simulink model "twoaxis_camera_gantry_start_work_project_Yejesh_final"  (R2025b)
settings: Solver=ode15s  StartTime=0.0  StopTime=60  MaxStep=1e-3  RelTol=1e-3  EnableMultiTasking=on
model workspace: external: MATLAB File gantryParams.m (data not in the file)
undefined symbols (not defined in the file): endSupport, endSupportZ, fractalcoef, leadScrew, leadScrewZ, rail, railZ, runner, runnerZ, X, Y, Z
libraries: sm_lib x81, nesl_utility x14, sm_linear_actuator_lib x14, fl_lib x6, slpidlib x2, mspsensorlib x1
(part 2 of 4)

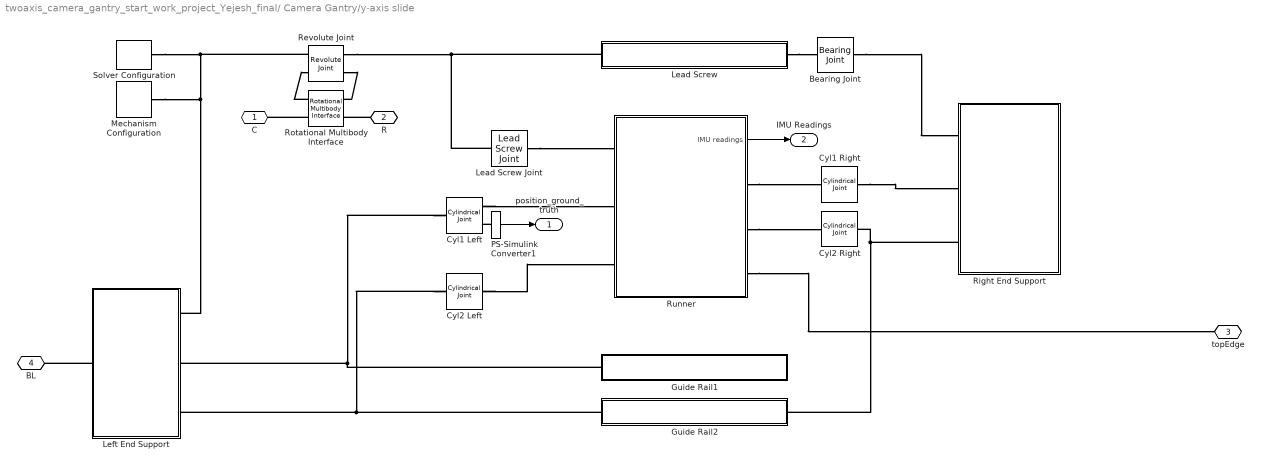
== system twoaxis_camera_gantry_start_work_project_Yejesh_final/	Camera Gantry/y-axis slide ==
  Bearing Joint : sm_lib/Joints/Bearing Joint  StatePerturbationForJacobian=1.0e-05  JointMode=Normal  CompositeWrenchDir=FollowerOnBase  CompositeWrenchFrame=BaseFrame  SenseConstraintForce=off  SenseConstraintTorque=off  SenseTotalForce=off  SenseTotalTorque=off  PzPositionTargetSpecify=off  PzPositionTargetPriority=High  PzPositionTargetValue=0  PzPositionTargetValueUnits=m  PzVelocityTargetSpecify=off  PzVelocityTargetPriority=High  PzVelocityTargetValue=0  PzVelocityTargetValueUnits=m/s  PzEquilibriumPosition=0  PzEquilibriumPositionUnits=m  PzSpringStiffness=0  PzSpringStiffnessUnits=N/m  PzDampingCoefficient=0  PzDampingCoefficientUnits=N/(m/s)  PzLowerLimitSpecify=off  PzLowerLimitBound=-1  PzLowerLimitBoundUnits=m  PzLowerLimitStiffness=1e6  PzLowerLimitStiffnessUnits=N/m  PzLowerLimitDamping=1e3  PzLowerLimitDampingUnits=N/(m/s)  PzLowerLimitTransitionRegionWidth=1e-4  PzLowerLimitTransitionRegionWidthUnits=m  PzUpperLimitSpecify=off  PzUpperLimitBound=1  PzUpperLimitBoundUnits=m  PzUpperLimitStiffness=1e6  PzUpperLimitStiffnessUnits=N/m  PzUpperLimitDamping=1e3  PzUpperLimitDampingUnits=N/(m/s)  PzUpperLimitTransitionRegionWidth=1e-4  PzUpperLimitTransitionRegionWidthUnits=m  PzTorqueActuationMode=NoTorque  PzMotionActuationMode=ComputedMotion  PzSensePosition=off  PzSenseVelocity=off  PzSenseAcceleration=off  PzSenseTorqueForce=off  PzSenseLowerLimitTorqueForce=off  PzSenseUpperLimitTorqueForce=off  RxPositionTargetSpecify=off  RxPositionTargetPriority=High  RxPositionTargetValue=0  RxPositionTargetValueUnits=deg  RxVelocityTargetSpecify=off  RxVelocityTargetPriority=High  RxVelocityTargetValue=0  RxVelocityTargetValueUnits=deg/s  RxEquilibriumPosition=0  RxEquilibriumPositionUnits=deg  RxSpringStiffness=0  RxSpringStiffnessUnits=N*m/deg  RxDampingCoefficient=0  RxDampingCoefficientUnits=N*m/(deg/s)  RxLowerLimitSpecify=off  RxLowerLimitBound=-90  RxLowerLimitBoundUnits=deg  RxLowerLimitStiffness=1e4  RxLowerLimitStiffnessUnits=N*m/deg  RxLowerLimitDamping=10  RxLowerLimitDampingUnits=N*m/(deg/s)  RxLowerLimitTransitionRegionWidth=0.1  RxLowerLimitTransitionRegionWidthUnits=deg  RxUpperLimitSpecify=off  RxUpperLimitBound=90  RxUpperLimitBoundUnits=deg  RxUpperLimitStiffness=1e4  RxUpperLimitStiffnessUnits=N*m/deg  RxUpperLimitDamping=10  RxUpperLimitDampingUnits=N*m/(deg/s)  RxUpperLimitTransitionRegionWidth=0.1  RxUpperLimitTransitionRegionWidthUnits=deg  RxTorqueActuationMode=NoTorque  RxMotionActuationMode=ComputedMotion  RxSensePosition=off  RxSenseVelocity=off  RxSenseAcceleration=off  RxSenseTorqueForce=off  RxSenseLowerLimitTorqueForce=off  RxSenseUpperLimitTorqueForce=off  RyPositionTargetSpecify=off  RyPositionTargetPriority=High  RyPositionTargetValue=0  RyPositionTargetValueUnits=deg  RyVelocityTargetSpecify=off  RyVelocityTargetPriority=High  RyVelocityTargetValue=0  RyVelocityTargetValueUnits=deg/s  RyEquilibriumPosition=0  RyEquilibriumPositionUnits=deg  RySpringStiffness=0  RySpringStiffnessUnits=N*m/deg  RyDampingCoefficient=0  RyDampingCoefficientUnits=N*m/(deg/s)  RyLowerLimitSpecify=off  RyLowerLimitBound=-90  RyLowerLimitBoundUnits=deg  RyLowerLimitStiffness=1e4  RyLowerLimitStiffnessUnits=N*m/deg  RyLowerLimitDamping=10  RyLowerLimitDampingUnits=N*m/(deg/s)  RyLowerLimitTransitionRegionWidth=0.1  RyLowerLimitTransitionRegionWidthUnits=deg  RyUpperLimitSpecify=off  RyUpperLimitBound=90  RyUpperLimitBoundUnits=deg  RyUpperLimitStiffness=1e4  RyUpperLimitStiffnessUnits=N*m/deg  RyUpperLimitDamping=10  RyUpperLimitDampingUnits=N*m/(deg/s)  RyUpperLimitTransitionRegionWidth=0.1  RyUpperLimitTransitionRegionWidthUnits=deg  RyTorqueActuationMode=NoTorque  RyMotionActuationMode=ComputedMotion  RySensePosition=off  RySenseVelocity=off  RySenseAcceleration=off  RySenseTorqueForce=off  RySenseLowerLimitTorqueForce=off  RySenseUpperLimitTorqueForce=off  RzPositionTargetSpecify=off  RzPositionTargetPriority=High  RzPositionTargetValue=0  RzPositionTargetValueUnits=deg  RzVelocityTargetSpecify=off  RzVelocityTargetPriority=High  RzVelocityTargetValue=0  RzVelocityTargetValueUnits=deg/s  RzEquilibriumPosition=0  RzEquilibriumPositionUnits=deg  RzSpringStiffness=0  RzSpringStiffnessUnits=N*m/deg  RzDampingCoefficient=b  RzDampingCoefficientUnits=N*m/(deg/s)  RzLowerLimitSpecify=off  RzLowerLimitBound=-90  RzLowerLimitBoundUnits=deg  RzLowerLimitStiffness=1e4  RzLowerLimitStiffnessUnits=N*m/deg  RzLowerLimitDamping=10  RzLowerLimitDampingUnits=N*m/(deg/s)  RzLowerLimitTransitionRegionWidth=0.1  RzLowerLimitTransitionRegionWidthUnits=deg  RzUpperLimitSpecify=off  RzUpperLimitBound=90  RzUpperLimitBoundUnits=deg  RzUpperLimitStiffness=1e4  RzUpperLimitStiffnessUnits=N*m/deg  RzUpperLimitDamping=10  RzUpperLimitDampingUnits=N*m/(deg/s)  RzUpperLimitTransitionRegionWidth=0.1  RzUpperLimitTransitionRegionWidthUnits=deg  RzTorqueActuationMode=NoTorque  RzMotionActuationMode=ComputedMotion  RzSensePosition=off  RzSenseVelocity=off  RzSenseAcceleration=off  RzSenseTorqueForce=off  RzSenseLowerLimitTorqueForce=off  RzSenseUpperLimitTorqueForce=off
  Cyl1 Left : sm_lib/Joints/Cylindrical Joint  StatePerturbationForJacobian=1.0e-05  JointMode=Normal  CompositeWrenchDir=FollowerOnBase  CompositeWrenchFrame=BaseFrame  SenseConstraintForce=off  SenseConstraintTorque=off  SenseTotalForce=off  SenseTotalTorque=off  RzPositionTargetSpecify=off  RzPositionTargetPriority=High  RzPositionTargetValue=0  RzPositionTargetValueUnits=deg  RzVelocityTargetSpecify=off  RzVelocityTargetPriority=High  RzVelocityTargetValue=0  RzVelocityTargetValueUnits=deg/s  RzEquilibriumPosition=0  RzEquilibriumPositionUnits=deg  RzSpringStiffness=0  RzSpringStiffnessUnits=N*m/deg  RzDampingCoefficient=0  RzDampingCoefficientUnits=N*m/(deg/s)  RzLowerLimitSpecify=off  RzLowerLimitBound=-90  RzLowerLimitBoundUnits=deg  RzLowerLimitStiffness=1e4  RzLowerLimitStiffnessUnits=N*m/deg  RzLowerLimitDamping=10  RzLowerLimitDampingUnits=N*m/(deg/s)  RzLowerLimitTransitionRegionWidth=0.1  RzLowerLimitTransitionRegionWidthUnits=deg  RzUpperLimitSpecify=off  RzUpperLimitBound=90  RzUpperLimitBoundUnits=deg  RzUpperLimitStiffness=1e4  RzUpperLimitStiffnessUnits=N*m/deg  RzUpperLimitDamping=10  RzUpperLimitDampingUnits=N*m/(deg/s)  RzUpperLimitTransitionRegionWidth=0.1  RzUpperLimitTransitionRegionWidthUnits=deg  RzTorqueActuationMode=NoTorque  RzMotionActuationMode=ComputedMotion  RzSensePosition=off  RzSenseVelocity=off  RzSenseAcceleration=off  RzSenseTorqueForce=off  RzSenseLowerLimitTorqueForce=off  RzSenseUpperLimitTorqueForce=off  PzPositionTargetSpecify=on  PzPositionTargetPriority=High  PzPositionTargetValue=position.bias  PzPositionTargetValueUnits=mm  PzVelocityTargetSpecify=off  PzVelocityTargetPriority=High  PzVelocityTargetValue=0  PzVelocityTargetValueUnits=m/s  PzEquilibriumPosition=0  PzEquilibriumPositionUnits=m  PzSpringStiffness=0  PzSpringStiffnessUnits=N/m  PzDampingCoefficient=0  PzDampingCoefficientUnits=N/(m/s)  PzLowerLimitSpecify=on  PzLowerLimitBound=endSupport.depth  PzLowerLimitBoundUnits=mm  PzLowerLimitStiffness=1e6  PzLowerLimitStiffnessUnits=N/m  PzLowerLimitDamping=1e3  PzLowerLimitDampingUnits=N/(m/s)  PzLowerLimitTransitionRegionWidth=1e-4  PzLowerLimitTransitionRegionWidthUnits=m  PzUpperLimitSpecify=on  PzUpperLimitBound=rail.length  PzUpperLimitBoundUnits=mm  PzUpperLimitStiffness=1e6  PzUpperLimitStiffnessUnits=N/m  PzUpperLimitDamping=1e3  PzUpperLimitDampingUnits=N/(m/s)  PzUpperLimitTransitionRegionWidth=1e-4  PzUpperLimitTransitionRegionWidthUnits=m  PzTorqueActuationMode=NoTorque  PzMotionActuationMode=ComputedMotion  PzSensePosition=on  PzSenseVelocity=off  PzSenseAcceleration=off  PzSenseTorqueForce=off  PzSenseLowerLimitTorqueForce=off  PzSenseUpperLimitTorqueForce=off
  Cyl1 Right : sm_lib/Joints/Cylindrical Joint  StatePerturbationForJacobian=1.0e-05  JointMode=Normal  CompositeWrenchDir=FollowerOnBase  CompositeWrenchFrame=BaseFrame  SenseConstraintForce=off  SenseConstraintTorque=off  SenseTotalForce=off  SenseTotalTorque=off  RzPositionTargetSpecify=off  RzPositionTargetPriority=High  RzPositionTargetValue=0  RzPositionTargetValueUnits=deg  RzVelocityTargetSpecify=off  RzVelocityTargetPriority=High  RzVelocityTargetValue=0  RzVelocityTargetValueUnits=deg/s  RzEquilibriumPosition=0  RzEquilibriumPositionUnits=deg  RzSpringStiffness=0  RzSpringStiffnessUnits=N*m/deg  RzDampingCoefficient=0  RzDampingCoefficientUnits=N*m/(deg/s)  RzLowerLimitSpecify=off  RzLowerLimitBound=-90  RzLowerLimitBoundUnits=deg  RzLowerLimitStiffness=1e4  RzLowerLimitStiffnessUnits=N*m/deg  RzLowerLimitDamping=10  RzLowerLimitDampingUnits=N*m/(deg/s)  RzLowerLimitTransitionRegionWidth=0.1  RzLowerLimitTransitionRegionWidthUnits=deg  RzUpperLimitSpecify=off  RzUpperLimitBound=90  RzUpperLimitBoundUnits=deg  RzUpperLimitStiffness=1e4  RzUpperLimitStiffnessUnits=N*m/deg  RzUpperLimitDamping=10  RzUpperLimitDampingUnits=N*m/(deg/s)  RzUpperLimitTransitionRegionWidth=0.1  RzUpperLimitTransitionRegionWidthUnits=deg  RzTorqueActuationMode=NoTorque  RzMotionActuationMode=ComputedMotion  RzSensePosition=off  RzSenseVelocity=off  RzSenseAcceleration=off  RzSenseTorqueForce=off  RzSenseLowerLimitTorqueForce=off  RzSenseUpperLimitTorqueForce=off  PzPositionTargetSpecify=off  PzPositionTargetPriority=High  PzPositionTargetValue=0  PzPositionTargetValueUnits=m  PzVelocityTargetSpecify=off  PzVelocityTargetPriority=High  PzVelocityTargetValue=0  PzVelocityTargetValueUnits=m/s  PzEquilibriumPosition=0  PzEquilibriumPositionUnits=m  PzSpringStiffness=0  PzSpringStiffnessUnits=N/m  PzDampingCoefficient=0  PzDampingCoefficientUnits=N/(m/s)  PzLowerLimitSpecify=off  PzLowerLimitBound=-410  PzLowerLimitBoundUnits=mm  PzLowerLimitStiffness=1e6  PzLowerLimitStiffnessUnits=N/m  PzLowerLimitDamping=1e3  PzLowerLimitDampingUnits=N/(m/s)  PzLowerLimitTransitionRegionWidth=1e-4  PzLowerLimitTransitionRegionWidthUnits=m  PzUpperLimitSpecify=off  PzUpperLimitBound=800  PzUpperLimitBoundUnits=mm  PzUpperLimitStiffness=1e6  PzUpperLimitStiffnessUnits=N/m  PzUpperLimitDamping=1e3  PzUpperLimitDampingUnits=N/(m/s)  PzUpperLimitTransitionRegionWidth=1e-4  PzUpperLimitTransitionRegionWidthUnits=m  PzTorqueActuationMode=NoTorque  PzMotionActuationMode=ComputedMotion  PzSensePosition=off  PzSenseVelocity=off  PzSenseAcceleration=off  PzSenseTorqueForce=off  PzSenseLowerLimitTorqueForce=off  PzSenseUpperLimitTorqueForce=off
  Cyl2 Left : sm_lib/Joints/Cylindrical Joint  StatePerturbationForJacobian=1.0e-05  JointMode=Normal  CompositeWrenchDir=FollowerOnBase  CompositeWrenchFrame=BaseFrame  SenseConstraintForce=off  SenseConstraintTorque=off  SenseTotalForce=off  SenseTotalTorque=off  RzPositionTargetSpecify=off  RzPositionTargetPriority=High  RzPositionTargetValue=0  RzPositionTargetValueUnits=deg  RzVelocityTargetSpecify=off  RzVelocityTargetPriority=High  RzVelocityTargetValue=0  RzVelocityTargetValueUnits=deg/s  RzEquilibriumPosition=0  RzEquilibriumPositionUnits=deg  RzSpringStiffness=0  RzSpringStiffnessUnits=N*m/deg  RzDampingCoefficient=0  RzDampingCoefficientUnits=N*m/(deg/s)  RzLowerLimitSpecify=off  RzLowerLimitBound=-90  RzLowerLimitBoundUnits=deg  RzLowerLimitStiffness=1e4  RzLowerLimitStiffnessUnits=N*m/deg  RzLowerLimitDamping=10  RzLowerLimitDampingUnits=N*m/(deg/s)  RzLowerLimitTransitionRegionWidth=0.1  RzLowerLimitTransitionRegionWidthUnits=deg  RzUpperLimitSpecify=off  RzUpperLimitBound=90  RzUpperLimitBoundUnits=deg  RzUpperLimitStiffness=1e4  RzUpperLimitStiffnessUnits=N*m/deg  RzUpperLimitDamping=10  RzUpperLimitDampingUnits=N*m/(deg/s)  RzUpperLimitTransitionRegionWidth=0.1  RzUpperLimitTransitionRegionWidthUnits=deg  RzTorqueActuationMode=NoTorque  RzMotionActuationMode=ComputedMotion  RzSensePosition=off  RzSenseVelocity=off  RzSenseAcceleration=off  RzSenseTorqueForce=off  RzSenseLowerLimitTorqueForce=off  RzSenseUpperLimitTorqueForce=off  PzPositionTargetSpecify=off  PzPositionTargetPriority=High  PzPositionTargetValue=250  PzPositionTargetValueUnits=mm  PzVelocityTargetSpecify=off  PzVelocityTargetPriority=High  PzVelocityTargetValue=0  PzVelocityTargetValueUnits=m/s  PzEquilibriumPosition=0  PzEquilibriumPositionUnits=m  PzSpringStiffness=0  PzSpringStiffnessUnits=N/m  PzDampingCoefficient=0  PzDampingCoefficientUnits=N/(m/s)  PzLowerLimitSpecify=on  PzLowerLimitBound=endSupport.depth  PzLowerLimitBoundUnits=mm  PzLowerLimitStiffness=1e6  PzLowerLimitStiffnessUnits=N/m  PzLowerLimitDamping=1e3  PzLowerLimitDampingUnits=N/(m/s)  PzLowerLimitTransitionRegionWidth=1e-4  PzLowerLimitTransitionRegionWidthUnits=m  PzUpperLimitSpecify=on  PzUpperLimitBound=rail.length  PzUpperLimitBoundUnits=mm  PzUpperLimitStiffness=1e6  PzUpperLimitStiffnessUnits=N/m  PzUpperLimitDamping=1e3  PzUpperLimitDampingUnits=N/(m/s)  PzUpperLimitTransitionRegionWidth=1e-4  PzUpperLimitTransitionRegionWidthUnits=m  PzTorqueActuationMode=NoTorque  PzMotionActuationMode=ComputedMotion  PzSensePosition=off  PzSenseVelocity=off  PzSenseAcceleration=off  PzSenseTorqueForce=off  PzSenseLowerLimitTorqueForce=off  PzSenseUpperLimitTorqueForce=off
  Cyl2 Right : sm_lib/Joints/Cylindrical Joint  StatePerturbationForJacobian=1.0e-05  JointMode=Normal  CompositeWrenchDir=FollowerOnBase  CompositeWrenchFrame=BaseFrame  SenseConstraintForce=off  SenseConstraintTorque=off  SenseTotalForce=off  SenseTotalTorque=off  RzPositionTargetSpecify=off  RzPositionTargetPriority=High  RzPositionTargetValue=0  RzPositionTargetValueUnits=deg  RzVelocityTargetSpecify=off  RzVelocityTargetPriority=High  RzVelocityTargetValue=0  RzVelocityTargetValueUnits=deg/s  RzEquilibriumPosition=0  RzEquilibriumPositionUnits=deg  RzSpringStiffness=0  RzSpringStiffnessUnits=N*m/deg  RzDampingCoefficient=0  RzDampingCoefficientUnits=N*m/(deg/s)  RzLowerLimitSpecify=off  RzLowerLimitBound=-90  RzLowerLimitBoundUnits=deg  RzLowerLimitStiffness=1e4  RzLowerLimitStiffnessUnits=N*m/deg  RzLowerLimitDamping=10  RzLowerLimitDampingUnits=N*m/(deg/s)  RzLowerLimitTransitionRegionWidth=0.1  RzLowerLimitTransitionRegionWidthUnits=deg  RzUpperLimitSpecify=off  RzUpperLimitBound=90  RzUpperLimitBoundUnits=deg  RzUpperLimitStiffness=1e4  RzUpperLimitStiffnessUnits=N*m/deg  RzUpperLimitDamping=10  RzUpperLimitDampingUnits=N*m/(deg/s)  RzUpperLimitTransitionRegionWidth=0.1  RzUpperLimitTransitionRegionWidthUnits=deg  RzTorqueActuationMode=NoTorque  RzMotionActuationMode=ComputedMotion  RzSensePosition=off  RzSenseVelocity=off  RzSenseAcceleration=off  RzSenseTorqueForce=off  RzSenseLowerLimitTorqueForce=off  RzSenseUpperLimitTorqueForce=off  PzPositionTargetSpecify=off  PzPositionTargetPriority=High  PzPositionTargetValue=0  PzPositionTargetValueUnits=m  PzVelocityTargetSpecify=off  PzVelocityTargetPriority=High  PzVelocityTargetValue=0  PzVelocityTargetValueUnits=m/s  PzEquilibriumPosition=0  PzEquilibriumPositionUnits=m  PzSpringStiffness=0  PzSpringStiffnessUnits=N/m  PzDampingCoefficient=0  PzDampingCoefficientUnits=N/(m/s)  PzLowerLimitSpecify=off  PzLowerLimitBound=-250  PzLowerLimitBoundUnits=mm  PzLowerLimitStiffness=1e6  PzLowerLimitStiffnessUnits=N/m  PzLowerLimitDamping=1e3  PzLowerLimitDampingUnits=N/(m/s)  PzLowerLimitTransitionRegionWidth=1e-4  PzLowerLimitTransitionRegionWidthUnits=m  PzUpperLimitSpecify=off  PzUpperLimitBound=250  PzUpperLimitBoundUnits=mm  PzUpperLimitStiffness=1e6  PzUpperLimitStiffnessUnits=N/m  PzUpperLimitDamping=1e3  PzUpperLimitDampingUnits=N/(m/s)  PzUpperLimitTransitionRegionWidth=1e-4  PzUpperLimitTransitionRegionWidthUnits=m  PzTorqueActuationMode=NoTorque  PzMotionActuationMode=ComputedMotion  PzSensePosition=off  PzSenseVelocity=off  PzSenseAcceleration=off  PzSenseTorqueForce=off  PzSenseLowerLimitTorqueForce=off  PzSenseUpperLimitTorqueForce=off
  Guide Rail1 : Subsystem  StatePerturbationForJacobian=1.0e-05  mask(Guide Rail){L=rail.length, R=rail.radius, rho=rail.density, color=rail.color}
      mask prompts: L "Length (mm)"; R "Radius (mm)"; rho "Density (kg/m^3)"; color "Color [r g b]"
      mask help:
      | This block models a guide rail of the linear actuator.
      |
      | The ports L and R correspond to the central points of the two end faces.
      mask DialogControl Container4 Prompt: Dimensions
      mask DialogControl Container5 Prompt: Material Properties
      mask Display:
      | image(fullfile(matlabroot,'toolbox','physmod','sm','smdemos','linear_actuator','images','sm_linear_actuator_guide_rail.png'));
      | port_label('lconn',1,'L');
      | port_label('rconn',1,'R');
  Guide Rail2 : Subsystem  StatePerturbationForJacobian=1.0e-05  mask(Guide Rail){L=rail.length, R=rail.radius, rho=rail.density, color=rail.color}
      mask prompts: L "Length (mm)"; R "Radius (mm)"; rho "Density (kg/m^3)"; color "Color [r g b]"
      mask help:
      | This block models a guide rail of the linear actuator.
      |
      | The ports L and R correspond to the central points of the two end faces.
      mask DialogControl Container4 Prompt: Dimensions
      mask DialogControl Container5 Prompt: Material Properties
      mask Display:
      | image(fullfile(matlabroot,'toolbox','physmod','sm','smdemos','linear_actuator','images','sm_linear_actuator_guide_rail.png'));
      | port_label('lconn',1,'L');
      | port_label('rconn',1,'R');
  Lead Screw : Subsystem  StatePerturbationForJacobian=1.0e-05  mask(Lead Screw){L=leadScrew.length, R=leadScrew.radius, rho=leadScrew.density, iColor=leadScrew.innerColor, oColor=leadScrew.outerColor}
      mask prompts: L "Length (mm)"; R "Radius (mm)"; rho "Density (kg/m^3)"; iColor "Inner Color [r g b]"; oColor "Outer Color [r g b]"
      mask help:
      | This block models the lead screw of the linear actuator.
      |
      | Ports L and R correspond to the central points of the two end faces.
      mask init:
      | x = 0.25*R;
      | 
      | theta = acos(x / R);
      | 
      | theta_arc = pi - 2 * theta;
      | 
      | theta_top_arc = linspace(theta, theta + theta_arc, 20);
      | theta_left_arc = linspace(theta + theta_arc, theta + pi, 20);
      | theta_bottom_arc = linspace(theta + pi, theta + pi + theta_arc, 20);
      | theta_right_arc = linspace(theta + pi + theta_arc, theta + 2*pi, 20);
      | 
      | left_section = [R*cos(theta_left_arc);
      |                   R*sin(theta_left_arc)]';
      | 
      | middle_section = [R*cos(theta_top_arc) R*cos(theta_bottom_arc);
      |                   R*sin(theta_top_arc) R*sin(theta_bottom_arc)]';
      | 
      | right_section = [R*cos(theta_right_arc);
      |                   R*sin(theta_right_arc)]';
      mask DialogControl Container4 Prompt: Dimensions
      mask DialogControl Container5 Prompt: Material Properties
      mask Display:
      | image(fullfile(matlabroot,'toolbox','physmod','sm','smdemos','linear_actuator','images','sm_linear_actuator_lead_screw.png'));
      | port_label('lconn',1,'L');
      | port_label('rconn',1,'R');
  Lead Screw Joint : sm_lib/Joints/Lead Screw Joint  StatePerturbationForJacobian=1.0e-05  JointMode=Normal  CompositeWrenchDir=FollowerOnBase  CompositeWrenchFrame=BaseFrame  SenseConstraintForce=off  SenseConstraintTorque=off  SenseTotalForce=off  SenseTotalTorque=off  Direction=RightHand  Lead=leadScrew.lead  LeadUnits=mm/rev  PositionTargetSpecify=off  PositionTargetPriority=High  PositionTargetRotationBased=off  PositionTargetRotationValue=0  PositionTargetRotationValueUnits=deg  PositionTargetTranslationValue=0  PositionTargetTranslationValueUnits=m  VelocityTargetSpecify=off  VelocityTargetPriority=High  VelocityTargetRotationBased=on  VelocityTargetRotationValue=0  VelocityTargetRotationValueUnits=deg/s  VelocityTargetTranslationValue=0  VelocityTargetTranslationValueUnits=m/s  SenseRotationPosition=off  SenseRotationVelocity=off  SenseRotationAcceleration=off  SenseTranslationPosition=off  SenseTranslationVelocity=off  SenseTranslationAcceleration=off
  Left End Support : Subsystem  StatePerturbationForJacobian=1.0e-05  mask(Left End Support){H=endSupport.height, W=endSupport.width, D=endSupport.depth, R1=endSupport.r_hole1, R2=endSupport.r_hole2and3, T=endSupport.bearingThickness, hole1_offset=endSupport.hole1_offset, hole2_offset=endSupport.hole2_offset, hole3_offset=endSupport.hole3_offset, rho=endSupport.density, sColor=endSupport.supportColor, bColor=endSupport.bearingColor}
      mask prompts: H "Height (mm)"; W "Width (mm)"; D "Depth (mm)"; R1 "Hole 1 Radius (mm)"; R2 "Holes 2 and 3 Radii (mm)"; T "Bearing Thickness (mm)"; hole1_offset "Hole 1 Offset [x y] (mm)"; hole2_offset "Hole 2 Offset [x y] (mm)"; hole3_offset "Hole 3 Offset [x y] (mm)"; rho "Density (mg/m^3)"; sColor "Support Color [r g b]"; bColor "Bearing Color [r g b]"
      mask help:
      | This block models the left end support of the linear actuator. The block comprises one End Support and one Hollow Cylinder which models the bearing on which the lead screw rotates.
      |
      | Ports H1, H2 and H3 correspond to the center point of each hole. Each is located on the rear face of the element.
      mask DialogControl Container4 Prompt: Dimensions
      mask DialogControl Container5 Prompt: Material Properties
      mask Display:
      | image(fullfile(matlabroot,'toolbox','physmod','sm','smdemos','linear_actuator','images','sm_linear_actuator_left_end_support.png'));
      | port_label('rconn',1,'H1');
      | port_label('rconn',2,'H2');
      | port_label('rconn',3,'H3');
  Mechanism Configuration : sm_lib/Utilities/Mechanism Configuration  StatePerturbationForJacobian=1.0e-05  UniformGravity=Constant  GravityVector=[0 0 -9.80665]  GravityVectorUnits=m/s^2  LinearizationDelta=0.001  JointModeTransitionNonlinearIterations=2
  PS-Simulink Converter1 : nesl_utility/PS-Simulink Converter  StatePerturbationForJacobian=1.0e-05  PhysicalDomain=network_engine_domain  SubClassName=ps_output  LeftPortType=input  RightPortType=output  PseudoPeriodic=off  Frequencies=[]  VectorFormat=1-D array  Unit=1  AffineConversion=off
  Revolute Joint : sm_lib/Joints/Revolute Joint  StatePerturbationForJacobian=1.0e-05  JointMode=Normal  CompositeWrenchDir=FollowerOnBase  CompositeWrenchFrame=BaseFrame  SenseConstraintForce=off  SenseConstraintTorque=off  SenseTotalForce=off  SenseTotalTorque=off  PositionTargetSpecify=off  PositionTargetPriority=High  PositionTargetValue=0  PositionTargetValueUnits=deg  VelocityTargetSpecify=off  VelocityTargetPriority=High  VelocityTargetValue=0  VelocityTargetValueUnits=deg/s  EquilibriumPosition=0  EquilibriumPositionUnits=deg  SpringStiffness=0  SpringStiffnessUnits=N*m/deg  DampingCoefficient=b  DampingCoefficientUnits=N*m/(deg/s)  LowerLimitSpecify=off  LowerLimitBound=-90  LowerLimitBoundUnits=deg  LowerLimitStiffness=1e4  LowerLimitStiffnessUnits=N*m/deg  LowerLimitDamping=10  LowerLimitDampingUnits=N*m/(deg/s)  LowerLimitTransitionRegionWidth=0.1  LowerLimitTransitionRegionWidthUnits=deg  UpperLimitSpecify=off  UpperLimitBound=90  UpperLimitBoundUnits=deg  UpperLimitStiffness=1e4  UpperLimitStiffnessUnits=N*m/deg  UpperLimitDamping=10  UpperLimitDampingUnits=N*m/(deg/s)  UpperLimitTransitionRegionWidth=0.1  UpperLimitTransitionRegionWidthUnits=deg  TorqueActuationMode=InputTorque  MotionActuationMode=ComputedMotion  SensePosition=off  SenseVelocity=on  SenseAcceleration=off  SenseTorqueForce=off  SenseLowerLimitTorqueForce=off  SenseUpperLimitTorqueForce=off
  Right End Support : Subsystem  StatePerturbationForJacobian=1.0e-05  mask{H=endSupport.height, W=endSupport.width, D=endSupport.depth, R1=endSupport.r_hole1, R2=endSupport.r_hole2and3, T=endSupport.bearingThickness, hole1_offset=endSupport.hole1_offset, hole2_offset=endSupport.hole2_offset, hole3_offset=endSupport.hole3_offset, rho=endSupport.density, sColor=endSupport.supportColor, bColor=endSupport.bearingColor}
      mask prompts: H "Height (mm)"; W "Width (mm)"; D "Depth (mm)"; R1 "Hole 1 Radius (mm)"; R2 "Holes 2 and 3 Radii (mm)"; T "Bearing Thickness (mm)"; hole1_offset "Hole 1 Offset [x y] (mm)"; hole2_offset "Hole 2 Offset [x y] (mm)"; hole3_offset "Hole 3 Offset [x y] (mm)"; rho "Density (mg/m^3)"; sColor "Support Color [r g b]"; bColor "Bearing Color [r g b]"
      mask help:
      | This block models the right end support of the linear actuator. The block comprises one End Support and one Hollow Cylinder which models the bearing on which the lead screw rotates.
      |
      | Ports H1, H2 and H3 correspond to the center point of each hole. Each is located on the rear face of the element.
      mask DialogControl Container4 Prompt: Dimensions
      mask DialogControl Container5 Prompt: Material Properties
      mask Display:
      | image(fullfile(matlabroot,'toolbox','physmod','sm','smdemos','linear_actuator','images','sm_linear_actuator_right_end_support.png'));
      | port_label('lconn',1,'H1');
      | port_label('lconn',2,'H2');
      | port_label('lconn',3,'H3');
  Rotational Multibody Interface : fl_lib/Mechanical/Multibody Interfaces/Rotational Multibody Interface
  Runner : Subsystem  StatePerturbationForJacobian=1.0e-05  mask(Runner){H=runner.height, W=runner.width, D=runner.depth, R1=runner.r_hole1, R2=runner.r_hole2and3, T=runner.bearingThickness, hole1_offset=runner.hole1_offset, hole2_offset=runner.hole2_offset, hole3_offset=runner.hole3_offset, rho=runner.density, rColor=runner.runnerColor, bColor=runner.bearingColor}
      mask prompts: H "Height (mm)"; W "Width (mm)"; D "Depth (mm)"; R1 "Hole 1 Radius (mm)"; R2 "Holes 2 and 3 Radii (mm)"; T "Bearing Thickness"; hole1_offset "Hole 1 Offset [x y] (mm)"; hole2_offset "Hole 2 Offset [x y] (mm)"; hole3_offset "Hole 3 Offset [x y] (mm)"; rho "Density (kg/m^3)"; rColor "Runner Color [r g b]"; bColor "Bearing Color [r g b]"
      mask help:
      | This block models the runner of the linear actuator. The block contains three Hollow Cylinder elements which model the bearings on which the runner slides and connect the runner to the lead screw.
      |
      | Port H1 corresponds to the lead screw connection and is located at the central point of hole 1.
      |
      | Ports H2L, H3L, H2R and H3R correspond to the connection points to the guide rails and are located at the center points of the holes on the front and rear faces.
      mask init:
      | hole_points = 40;
      | 
      | qHole1 = linspace(pi/2, pi/2-2*pi, hole_points);
      | r1 = R1+T;
      | hole1 = [r1*cos(qHole1);
      |          r1*sin(qHole1)+hole1_offset(2)]';
      | 
      | qHole2 = linspace(0, -2*pi, hole_points);
      | r2 = R2+T;
      | hole2 = [r2*cos(qHole2)+hole2_offset(1); 
      |          r2*sin(qHole2)+hole2_offset(2)]';
      | 
      | qHole3 = linspace(pi, -pi, hole_points);
      | hole3 = [r2*cos(qHole3)+hole3_offset(1); 
      |          r2*sin(qHole3)+hole3_offset(2)]';
      | 
      | extrusion_points = [ 0     0;
      |                      0.5*W 0;
      |                      0.5*W hole2_offset(2);
      |                      hole2;
      |                      0.5*W hole2_offset(2);
      |                      0.5*W H;
      |                      0     H;
      |                      hole1;
      |                      0     H;
      |                     -0.5*W H;
      |                     -0.5*W hole3_offset(2);
      |                      hole3;
      |                     -0.5*W hole3_offset(2);
      |                     -0.5*W 0];
      mask DialogControl Container4 Prompt: Runner Dimensions
      mask DialogControl Container9 Prompt: Material Properties
      mask Display:
      | image(fullfile(matlabroot,'toolbox','physmod','sm','smdemos','linear_actuator','images','sm_linear_actuator_runner.png'));
      | port_label('lconn',1,'H1');
      | port_label('lconn',2,'H2L');
      | port_label('lconn',3,'H3L');
      | port_label('rconn',1,'H2R');
      | port_label('rconn',2,'H3R');
  Solver Configuration : nesl_utility/Solver Configuration  StatePerturbationForJacobian=1.0e-05  PhysicalDomain=network_engine_domain  SubClassName=solver  LeftPortType=input  RightPortType=generic  Tones=[]  Harmonics=[]  SimulateNoise=off  Profile=off  UseLocalSampling=off  EnableSwitchedLinearOptims=on  FrequencyDomain=off  UseCCode=off  RelTol=0.001  AbsTol=1e-06  MinStep=1e-09  ToWorkspace=off  RevertToSquareIcSolve=off  NumHomotopyIterations=100  PhasorMode=off  PhasorModeNumHarmonics=1  ConsistencySolver=NEWTON_FTOL  IndexReductionMethod=DerivativeReplacement  DoDC=off  ResidualTolerance=1e-09  ConsistencyTolSource=GLOBAL  ConsistencyAbsTol=0.001  ConsistencyRelTol=0.001  ConsistencyTolFactor=0.001  UseLocalSolver=off  LocalSolverChoice=NE_BACKWARD_EULER_ADVANCER  ResolveIndetEquations=on  FunctionEvalNumThread=1  LocalSolverSampleTime=0.001  DoFixedCost=off  MaxNonlinIter=3  MaxModeIter=2  ComputeImpulses=off  ImpulseIterations=2  LinearAlgebra=Sparse  LinearAlgebraNumThread=0  EquationFormulation=NE_TIME_EF  DelaysMemoryBudget=1024  AutomaticFiltering=on  FilteringTimeConstant=0.001  PartitionStorageMethod=AS_NEEDED  PartitionMemoryBudget=1024  PartitionMethod=FAST  MultibodyUseLocalSolver=off  MultibodyLocalSolverChoice=ODE1  MultibodyLocalSolverSampleTime=0.001
  C : PMIOPort  Side=Left
  R : PMIOPort  Port=2  Side=Left
  topEdge : PMIOPort  Port=3  Side=Right
  BL : PMIOPort  Port=4  Side=Right
  position_ground_truth : Outport
  IMU Readings : Outport  Port=2
  wires:
  PS-Simulink Converter1/1 -> position_ground_truth/1
  Runner/1(IMU readings) -> IMU Readings/1
  connections:
  Rotational Multibody Interface/LConn2 -- C/RConn1
  PS-Simulink Converter1/LConn1 -- Cyl1 Left/RConn2
  Revolute Joint/LConn1 -- Left End Support/RConn1 -- Mechanism Configuration/RConn1 -- Solver Configuration/RConn1
  Guide Rail2/LConn1 -- Cyl2 Left/LConn1 -- Left End Support/RConn3
  Revolute Joint/RConn2 -- Rotational Multibody Interface/RConn1
  Revolute Joint/RConn1 -- Lead Screw/LConn1 -- Lead Screw Joint/LConn1
  Right End Support/LConn3 -- Cyl2 Right/LConn1 -- Guide Rail2/RConn1
  Runner/RConn3 -- topEdge/RConn1
  Guide Rail1/LConn1 -- Cyl1 Left/LConn1 -- Left End Support/RConn2
  Cyl2 Left/RConn1 -- Runner/LConn3
  Bearing Joint/LConn1 -- Right End Support/LConn1
  Runner/RConn2 -- Cyl2 Right/RConn1
  Cyl1 Left/RConn1 -- Runner/LConn2
  Runner/RConn1 -- Cyl1 Right/RConn1
  Lead Screw Joint/RConn1 -- Runner/LConn1
  R/RConn1 -- Rotational Multibody Interface/RConn2
  Lead Screw/RConn1 -- Bearing Joint/RConn1
  Cyl1 Right/LConn1 -- Right End Support/LConn2
  Rotational Multibody Interface/LConn1 -- Revolute Joint/LConn2
  Left End Support/LConn1 -- BL/RConn1
